simulink model "CruiseControl_P_Controller"  (R2026a)
settings: Solver=ode45  StopTime=20  MaxStep=0.01
undefined symbols (not defined in the file): Kp
settings Model: Creator=YASHRK  LastModifiedBy=YASHRK

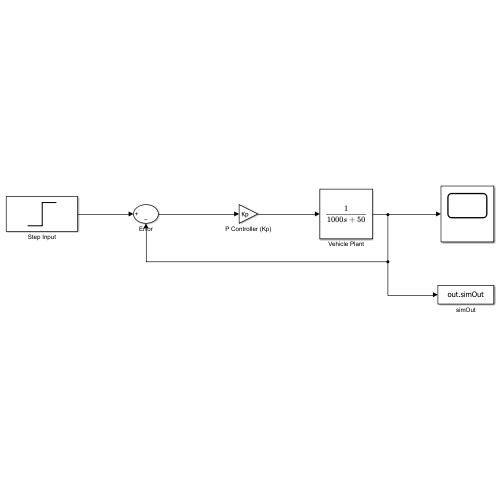
[thumbnail: Simulink's stored preview of the top-level diagram]
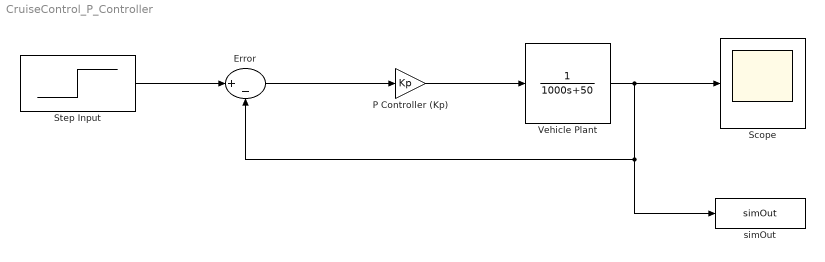
== system CruiseControl_P_Controller ==
  Error : Sum  Inputs=|+-
  P Controller (Kp) : Gain  Gain=Kp
  Scope : Scope
      settings: ActiveDisplayYMinimum=-0.33496370728607205  ActiveDisplayYMaximum=1.1878722479696098
  Step Input : Step  Time=0  SampleTime=0
  Vehicle Plant : TransferFcn  Denominator=[1000 50]
  simOut : ToWorkspace  VariableName=simOut  SaveFormat=Structure With Time  SampleTime=-1
  wires:
  Step Input/1 -> Error/1
  Error/1 -> P Controller (Kp)/1
  P Controller (Kp)/1 -> Vehicle Plant/1
  Vehicle Plant/1 -> simOut/1, Error/2, Scope/1
